simulink library "DCL"  (R2018b)
settings: Solver=VariableStepAuto  StartTime=0.0  StopTime=10.0  RelTol=1e-3
undefined symbols (not defined in the file or in its folder): Uc_max, Uc_min
libraries: simulink x11
settings Model: Creator=a0741273  LastModifiedBy=a0741273
settings SFSimCC: SimUseLocalCustomCode=off
settings RTWCC: RTWUseLocalCustomCode=off

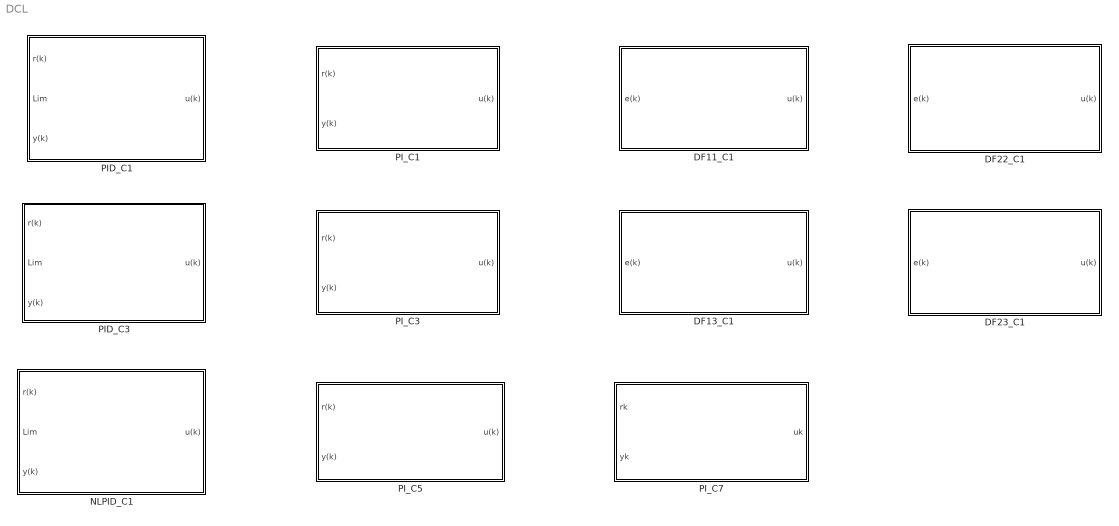
== system DCL ==
  DF11_C1 : Subsystem  TreatAsAtomicUnit=on  SystemSampleTime=T  mask{b0=1, b1=0, a1=0, T=0.001}
      mask prompts: b0 "Coefficient b0"; b1 "Coefficient b1"; a1 "Coefficient a1"; T "Sample period in seconds"
      mask Help:
      | The DF11_C1 block provides a functional model of a first order discrete "direct form 1" compensator in the C2000 Digital Control Library (DCL).
      | 
      | The control law is:
      | u(k) = b0*e(k) + b1*e(k-1) - a1*u(k-1)
      | 
      | T = The sample period (controller update rate) in seconds.
      | 
      | Refer to the DCL User's Guide for further information about this controller.  The model is not configured to support code generation.
      mask DialogControl DescTextVar Prompt: DF11_C1 Controller Parameters
      mask Display: disp('DF11_C1')
  DF13_C1 : Subsystem  TreatAsAtomicUnit=on  mask{b0=1, b1=0, b2=0, b3=0, a1=0, a2=0, a3=0, T=0.001}
      mask prompts: b0 "Coefficient b0"; b1 "Coefficient b1"; b2 "Coefficient b2"; b3 "Coefficient b3"; a1 "Coefficient a1"; a2 "Coefficient a2"; a3 "Coefficient a3"; T "Sample period in seconds"
      mask Help:
      | The DF13_C1 block provides a functional model of a third order discrete "direct form 1" compensator in the C2000 Digital Control Library (DCL).
      | 
      | The control law is:
      | u(k) = b0*e(k) + b1*e(k-1) + b2*e(k-2) + b3*e(k-3) - a1*u(k-1) - a2*u(k-2) - a3*u(k-3)
      | 
      | T = The sample period (controller update rate) in seconds.
      | 
      | Refer to the DCL User's Guide for further information about this controller.  The model is not configured to support code generation.
      mask DialogControl DescTextVar Prompt: DF13_C1 Controller Parameters
      mask DialogControl T Tooltip: Enter sample period in seconds
      mask Display: disp('DF13_C1')
  DF22_C1 : Subsystem  TreatAsAtomicUnit=on  SystemSampleTime=T  mask{b0=1, b1=0, b2=0, a1=0, a2=0, T=0.001}
      mask prompts: b0 "Coefficient b0"; b1 "Coefficient b1"; b2 "Coefficient b2"; a1 "Coefficient a1"; a2 "Coefficient a2"; T "Sample period in seconds"
      mask Help:
      | The DF22_C1 block provides a functional model of a second order discrete "direct form 2" compensator in the C2000 Digital Control Library (DCL).
      | 
      | The control law is:
      | u(k) = b0*e(k) + b1*e(k-1) + b2*e(k-2) - a1*u(k-1) - a2*u(k-2)
      | 
      | T = The sample period (controller update rate) in seconds.
      | 
      | Refer to the DCL User's Guide for further information about this controller.  The model is not configured to support code generation.
      mask DialogControl DescTextVar Prompt: CF22_C1 Controller Parameters
      mask Display: disp('DF22_C1')
  DF23_C1 : Subsystem  TreatAsAtomicUnit=on  mask{b0=1, b1=0, b2=0, b3=0, a1=0, a2=0, a3=0, T=0.001}
      mask prompts: b0 "Coefficient b0"; b1 "Coefficient b1"; b2 "Coefficient b2"; b3 "Coefficient b3"; a1 "Coefficient a1"; a2 "Coefficient a2"; a3 "Coefficient a3"; T "Sample period in seconds"
      mask Help:
      | he DF23_C1 block provides a functional model of a third order discrete "direct form 2" compensator in the C2000 Digital Control Library (DCL).
      | 
      | The control law is:
      | u(k) = b0*e(k) + b1*e(k-1) + b2*e(k-2) + b3*e(k-3) - a1*u(k-1) - a2*u(k-2) - a3*u(k-3)
      | 
      | T = The sample period (controller update rate) in seconds.
      | 
      | Refer to the DCL User's Guide for further information about this controller.  The model is not configured to support code generation.
      mask DialogControl DescTextVar Prompt: DF23_C1 Controller Parameters
      mask Display: disp('DF23_C1')
  NLPID_C1 : Subsystem  TreatAsAtomicUnit=on  SystemSampleTime=T  mask{Kp=1, Ki=0, Kd=0, alpha_p=1, alpha_i=1, alpha_d=1, delta_p=0.1, delta_i=0.1, delta_d=0.1, fc=100, Umax=1, Umin=-1, T=0.001}
      mask prompts: Kp "Linear Proportional Gain (Kp)"; Ki "Linear Integral Gain (Ki)"; Kd "Linear Derivative Gain (Kd)"; alpha_p "P-path Non-linear Coefficient (alpha_p)"; alpha_i "I-path Non-linear Coefficient (alpha_i)"; alpha_d "D-path Non-linear Coefficient (alpha_d)"; delta_p "P-path Linear Semi-width (delta_p)"; delta_i "I-path Linear Semi-width (delta_i)"; delta_d "D-path Linear Semi-width (delta_d)"; fc "Derivative Filter Bandwidth in Hz"; Umax "Output Clamp Upper Limit (Umax)"; Umin "Output Clamp Lower Limit (Umin)"; T "Sample Period in seconds"
      mask help: C2000 Digital Control Library blocks
      mask init:
      | tau = 1 / (2*pi*fc);
      | c1 = 2 / (T + 2*tau);
      | c2 = (T - 2*tau) / (T + 2*tau);
      | 
      | gamma_p = 1 / (delta_p^(1 - alpha_p));
      | gamma_i = 1 / (delta_i^(1 - alpha_i));
      | gamma_d = 1 / (delta_d^(1 - alpha_d));
      mask Help:
      | The NLPID_C1 block provides a functional model of the non-linear PID controller in the C2000 Digital Control Library (DCL).
      | 
      | Kp = Linear proportional gain
      | Ki = Linear integral gain
      | Kd = Linear derivative gain
      | alpha_p = P-path non-linear exponent
      | alpha_i = I-path non-linear exponent
      | alpha_d = D-path non-linear exponent
      | delta_p = P-path linearized semi-width
      | delta_i = I-path linearized semi-width
      | delta_d = D-path linearized semi-width
      | Umax = Output clamp upper limit
      | Umin = Output clamp lower limit
      | 
      | Refer to the DCL User's Guide for further information on this controller.  The model is not configured to support code generation.
      mask DialogControl DescTextVar Prompt: NLPID_C1 Controller Parameters
      mask Display:
      | disp('NLPID_C1')
      | % image('C:\Aa07\projects\DCL\models\SLOGO.jpg')
  PID_C1 : Subsystem  TreatAsAtomicUnit=on  SystemSampleTime=T  mask{Kp=1, Ki=0, Kd=0, Kr=1, fc=100, Umax=1, Umin=-1, T=0.001}
      mask prompts: Kp "Proportional Gain (Kp)"; Ki "Integral Gain (Ki)"; Kd "Derivative Gain (Kd)"; Kr "Set-point Gain (Kr)"; fc "Derivative Filter Bandwidth in Hz (fc)"; Umax "Output Clamp Upper Limit (Umax)"; Umin "Output Clamp Lower Limit (Umin)"; T "Sample Period in seconds (T)"
      mask init:
      | tau = 1 / (2*pi*fc);
      | c1 = 2 / (T + 2*tau);
      | c2 = (T - 2*tau) / (T + 2*tau);
      mask Help:
      | The PID_C1 block provides a functional model of the series form linear PID controller in the C2000 Digital Control Library (DCL).
      | 
      | Kp = The proportional path gain.
      | 
      | Ki = The integral path gain scaled by the sample period (T).
      | 
      | Kd = The derivative path gain.  Sample period enters the control law through the derivative filter coefficients, so is not accounted for in Kd.
      | 
      | Kr = The set-point weighting factor.
      | 
      | fc = The -3dB bandwidth of the derivative filter in Hz.  This is used to compute the derivative filter coefficients c1 & c2.
      | 
      | Umax = The upper limit of the output clamp.
      | 
      | Umin = The lower limit of the output clamp.
      | 
      | T = The sample period (controller update rate) in seconds.
      | 
      | Refer to the DCL User's Guide for further information about this controller.  The model is not configured to support code generation.
      mask DialogControl DescTextVar Prompt: PID_C1 Controller Parameters
      mask Display: disp('PID_C1')
  PID_C3 : Subsystem  TreatAsAtomicUnit=on  SystemSampleTime=T  mask{Kp=1, Ki=0, Kd=0, fc=100, Umax=1, Umin=-1, T=0.001}
      mask prompts: Kp "Proportional Gain (Kp)"; Ki "Integral Gain (Ki)"; Kd "Derivative Gain (Kd)"; fc "Derivative Filter Bandwidth in Hz (fc)"; Umax "Output Clamp Upper Limit (Umax)"; Umin "Output Clamp Lower Limit (Umin)"; T "Sample Period in seconds (T)"
      mask init:
      | tau = 1 / (2*pi*fc);
      | c1 = 2 / (T + 2*tau);
      | c2 = (T - 2*tau) / (T + 2*tau);
      mask Help:
      | The PID_C3 block provides a functional model of the parallel form linear PID controller in the C2000 Digital Control Library (DCL).
      | 
      | Kp = The proportional path gain.
      | 
      | Ki = The integral path gain scaled by the sample period (T).
      | 
      | Kd = The derivative path gain.  Sample period enters the control law through the derivative filter coefficients, so is not accounted for in Kd.
      | 
      | fc = The -3dB bandwidth of the derivative filter in Hz.  This is used to compute the derivative filter coefficients c1 & c2.
      | 
      | Umax = The upper limit of the output clamp.
      | 
      | Umin = The lower limit of the output clamp.
      | 
      | T = The sample period (controller update rate) in seconds.
      | 
      | Refer to the DCL User's Guide for further information about this controller.  The model is not configured to support code generation.
      mask DialogControl DescTextVar Prompt: PID_C3 Controller Parameters
      mask Display: disp('PID_C3')
  PI_C1 : Subsystem  TreatAsAtomicUnit=on  SystemSampleTime=T  mask{Kp=1, Ki=0, Umax=1, Umin=-1, T=0.001}
      mask prompts: Kp "Proportional Gain (Kp)"; Ki "Integral Gain (Ki)"; Umax "Output Clamp Upper Limit (Umax)"; Umin "Output Clamp Upper Limit (Umin)"; T "Sample period in seconds"
      mask Help:
      | The PI_C1 block provides a functional model of the series form linear PI controller in the C2000 Digital Control Library (DCL).
      | 
      | Kp = The proportional path gain.
      | 
      | Ki = The integral path gain scaled by the sample period (T).
      | 
      | Umax = The upper limit of the output clamp.
      | 
      | Umin = The lower limit of the output clamp.
      | 
      | T = The sample period (controller update rate) in seconds.
      | 
      | Refer to the DCL User's Guide for further information about this controller.  The model is not configured to support code generation.
      mask DialogControl DescTextVar Prompt: PI_C3 Controller Parameters
      mask Display: disp('PI_C1')
  PI_C3 : Subsystem  TreatAsAtomicUnit=on  SystemSampleTime=T  mask{Kp=1, Ki=0, Umax=1, Umin=-1, T=0.001}
      mask prompts: Kp "Proportional Gain (Kp)"; Ki "Integral Gain (Ki)"; Umax "Output Clamp Upper Limit (Umax)"; Umin "Output Clamp Lower Limit (Umin)"; T "Sample period in seconds"
      mask Help:
      | The PI_C3 block provides a functional model of the parallel form linear PI controller in the C2000 Digital Control Library (DCL).
      | 
      | Kp = The proportional path gain.
      | 
      | Ki = The integral path gain scaled by the sample period (T).
      | 
      | Umax = The upper limit of the output clamp.
      | 
      | Umin = The lower limit of the output clamp.
      | 
      | T = The sample period (controller update rate) in seconds.
      | 
      | Refer to the DCL User's Guide for further information about this controller.  The model is not configured to support code generation.
      mask DialogControl DescTextVar Prompt: PI_C3 Controller Parameters
      mask Display: disp('PI_C3')
  PI_C5 : Subsystem  TreatAsAtomicUnit=on  SystemSampleTime=T  mask{Kp=1, Ki=0, Umax=1, Umin=-1, Imax=1, Imin=-1, T=0.001}
      mask prompts: Kp "Proportional Gain (Kp)"; Ki "Integral Gain (Ki)"; Umax "Output Clamp Upper Limit (Umax)"; Umin "Output Clamp Lower Limit (Umin)"; Imax "Integrator Clamp Upper Limit (Imax)"; Imin "Integrator Clamp Lower Limit (Imin)"; T "Sample period in seconds"
      mask Help:
      | The PI_C5 block provides a functional model of the parallel form linear PI controller in the C2000 Digital Control Library (DCL).  This controller comprises separate integral path and output clamp limits and employs improved, though less cycle efficient, anti-windup reset logic.
      | 
      | Kp = The proportional path gain.
      | 
      | Ki = The integral path gain scaled by the sample period (T).
      | 
      | Umax = The upper limit of the output clamp.
      | 
      | Umin = The lower limit of the output clamp.
      | 
      | Imax = The upper limit of the integrator clamp.
      | 
      | Imin = The lower limit of the integrator clamp.
      | 
      | T = The sample period (controller update rate) in seconds.
      | 
      | Refer to the DCL User's Guide for further information about this controller.  The model is not configured to support code generation.
      mask DialogControl DescTextVar Prompt: PI_C5 Controller Parameters
      mask Display: disp('PI_C5')
  PI_C7 : Subsystem  mask{Kp=1, Ki=0, Umax=1, Umin=-1, T=0.001}
      mask prompts: Kp "Proportional Gain (Kp)"; Ki "Integral Gain (Ki)"; Umax "Output clamp Upper Limit (Umax)"; Umin "Output Clamp Lower Limit (Umin)"; T "Sample Rate in Seconds"
      mask Help:
      | The PI_C7 block provides a functional model of the series form linear PI controller with Tustin integrator in the C2000 Digital Control Library (DCL).  The model is functionally similar to the PI_C6 and PI_C7 controllers.
      | 
      | Kp = The proportional path gain.
      | 
      | Ki = The integral path gain scaled by the sample period (T).
      | 
      | Umax = The upper limit of the output clamp.
      | 
      | Umin = The lower limit of the output clamp.
      | 
      | T = The sample period (controller update rate) in seconds.
      | 
      | Refer to the DCL User's Guide for further information about this controller.  The model is not configured to support code generation.
      mask DialogControl DescTextVar Prompt: PI_C7 Controller Parameters
      mask Display: disp('PI_C7')

== system DCL/DF11_C1 ==
  e(k) : Inport
  Gain : Gain  Gain=b0
  Gain1 : Gain  Gain=b1
  Gain2 : Gain  Gain=a1
  Sum : Sum  Inputs=+|-
  Sum1 : Sum  Inputs=++|
  Unit Delay : UnitDelay  SampleTime=-1
  Unit Delay5 : UnitDelay  SampleTime=-1
  u(k) : Outport
  wires:
  Gain/1 -> Sum/1
  Unit Delay/1 -> Gain1/1
  e(k)/1 -> Gain/1, Unit Delay/1
  Unit Delay5/1 -> Gain2/1
  Gain1/1 -> Sum1/1
  Sum/1 -> Sum1/2
  Sum1/1 -> Unit Delay5/1, u(k)/1
  Gain2/1 -> Sum/2

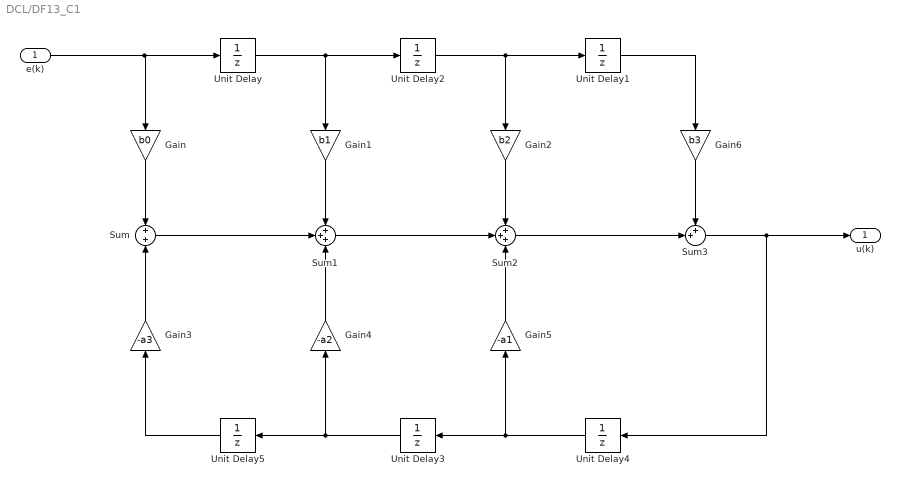
== system DCL/DF13_C1 ==
  e(k) : Inport
  Gain : Gain  Gain=b0
  Gain1 : Gain  Gain=b1
  Gain2 : Gain  Gain=b2
  Gain3 : Gain  Gain=-a3
  Gain4 : Gain  Gain=-a2
  Gain5 : Gain  Gain=-a1
  Gain6 : Gain  Gain=b3
  Sum : Sum  Inputs=+|+
  Sum1 : Sum  Inputs=+++
  Sum2 : Sum  Inputs=+++
  Sum3 : Sum  Inputs=++|
  Unit Delay{,1..5} (6 alike) : UnitDelay  SampleTime=-1
  "u(k) " : Outport
  wires:
  e(k)/1 -> Gain/1, Unit Delay/1
  Unit Delay/1 -> Gain1/1, Unit Delay2/1
  Unit Delay2/1 -> Gain2/1, Unit Delay1/1
  Unit Delay4/1 -> Gain5/1, Unit Delay3/1
  Unit Delay3/1 -> Gain4/1, Unit Delay5/1
  Gain/1 -> Sum/1
  Gain1/1 -> Sum1/1
  Gain2/1 -> Sum2/1
  Sum/1 -> Sum1/2
  Sum1/1 -> Sum2/2
  Gain3/1 -> Sum/2
  Gain4/1 -> Sum1/3
  Gain5/1 -> Sum2/3
  Unit Delay1/1 -> Gain6/1
  Gain6/1 -> Sum3/1
  Sum2/1 -> Sum3/2
  Unit Delay5/1 -> Gain3/1
  Sum3/1 -> "u(k) "/1, Unit Delay4/1

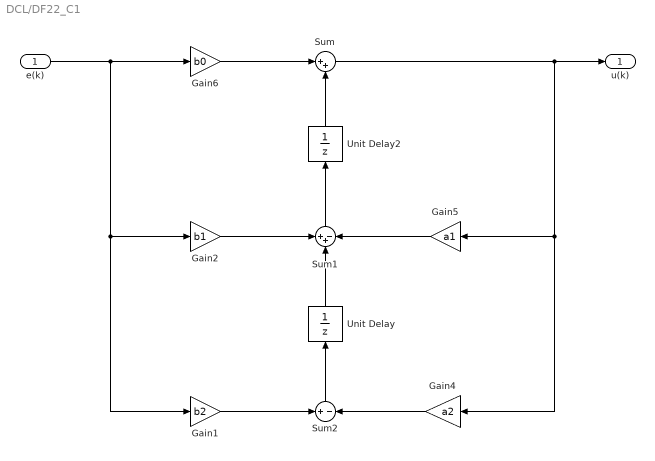
== system DCL/DF22_C1 ==
  e(k) : Inport
  Gain1 : Gain  Gain=b2
  Gain2 : Gain  Gain=b1
  Gain4 : Gain  Gain=a2
  Gain5 : Gain  Gain=a1
  Gain6 : Gain  Gain=b0
  Sum : Sum  Inputs=|++
  Sum1 : Sum  Inputs=++-
  Sum2 : Sum  Inputs=+|-
  Unit Delay : UnitDelay  SampleTime=-1
  Unit Delay2 : UnitDelay  SampleTime=-1
  "u(k) " : Outport
  wires:
  Gain2/1 -> Sum1/1
  Unit Delay/1 -> Sum1/2
  Sum1/1 -> Unit Delay2/1
  Unit Delay2/1 -> Sum/2
  Gain5/1 -> Sum1/3
  Gain4/1 -> Sum2/2
  Sum2/1 -> Unit Delay/1
  Gain1/1 -> Sum2/1
  e(k)/1 -> Gain2/1, Gain1/1, Gain6/1
  Gain6/1 -> Sum/1
  Sum/1 -> Gain4/1, Gain5/1, "u(k) "/1

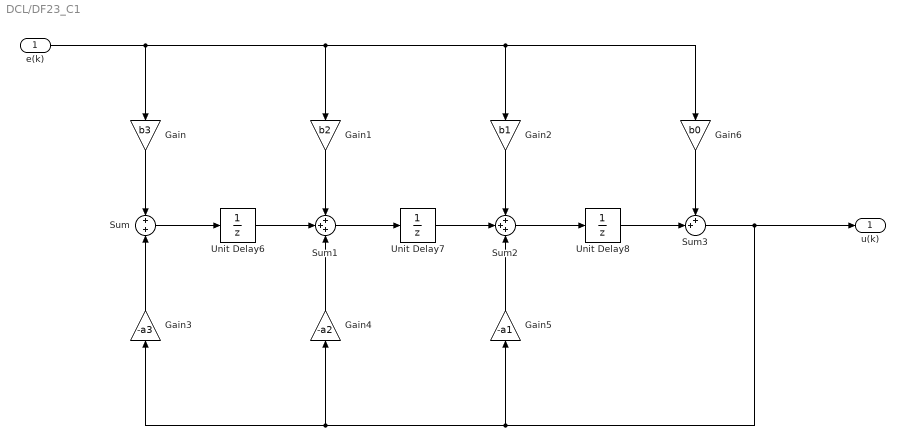
== system DCL/DF23_C1 ==
  e(k) : Inport
  Gain : Gain  Gain=b3
  Gain1 : Gain  Gain=b2
  Gain2 : Gain  Gain=b1
  Gain3 : Gain  Gain=-a3
  Gain4 : Gain  Gain=-a2
  Gain5 : Gain  Gain=-a1
  Gain6 : Gain  Gain=b0
  Sum : Sum  Inputs=+|+
  Sum1 : Sum  Inputs=+++
  Sum2 : Sum  Inputs=+++
  Sum3 : Sum  Inputs=++|
  Unit Delay6 : UnitDelay  SampleTime=-1
  Unit Delay7 : UnitDelay  SampleTime=-1
  Unit Delay8 : UnitDelay  SampleTime=-1
  "u(k) " : Outport
  wires:
  Gain/1 -> Sum/1
  Gain1/1 -> Sum1/1
  Gain2/1 -> Sum2/1
  Gain3/1 -> Sum/2
  Gain4/1 -> Sum1/3
  Gain5/1 -> Sum2/3
  e(k)/1 -> Gain/1, Gain6/1, Gain2/1, Gain1/1
  Gain6/1 -> Sum3/1
  Sum3/1 -> Gain3/1, Gain4/1, Gain5/1, "u(k) "/1
  Unit Delay8/1 -> Sum3/2
  Sum2/1 -> Unit Delay8/1
  Unit Delay7/1 -> Sum2/2
  Sum1/1 -> Unit Delay7/1
  Unit Delay6/1 -> Sum1/2
  Sum/1 -> Unit Delay6/1

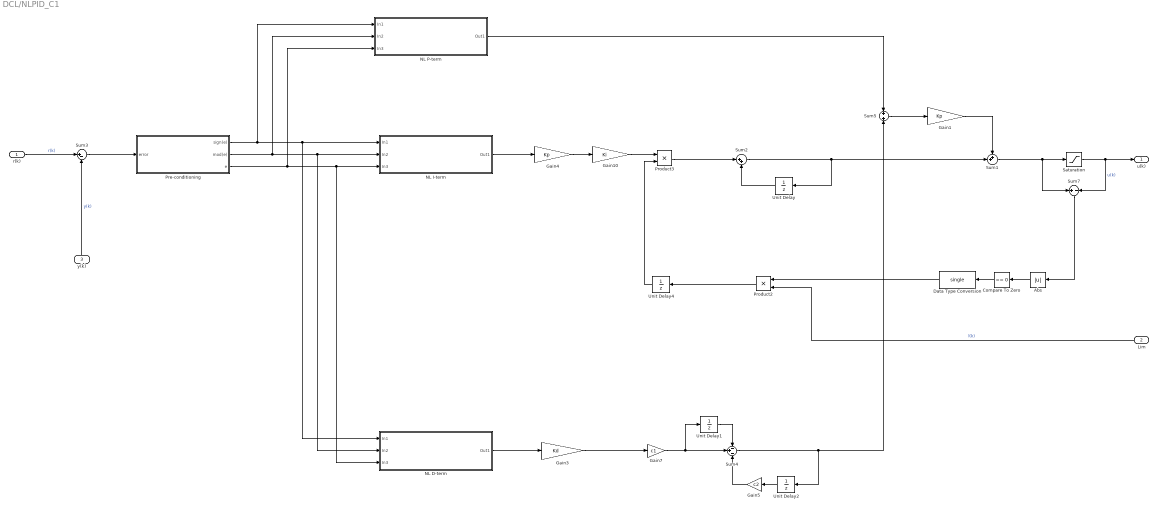
== system DCL/NLPID_C1 ==
  r(k) : Inport  OutDataTypeStr=single  SampleTime=T
  Lim : Inport  Port=2  OutDataTypeStr=single  SampleTime=T  LockScale=on
  y(k) : Inport  Port=3  OutDataTypeStr=single  SampleTime=T  LockScale=on
  Abs : Abs
  Compare To Zero : simulink/Logic and Bit Operations/Compare To Zero  relop===  OutDataTypeStr=boolean
  Data Type Conversion : DataTypeConversion  OutDataTypeStr=single
  Gain1 : Gain  Gain=Kp
  Gain10 : Gain  Gain=Ki
  Gain3 : Gain  Gain=Kd
  Gain4 : Gain  Gain=Kp
  Gain5 : Gain  Gain=c2  ParamDataTypeStr=single  OutDataTypeStr=single  LockScale=on
  Gain7 : Gain  Gain=c1
  NL D-term : Subsystem
  NL I-term : Subsystem
  NL P-term : Subsystem
  Pre-conditioning : Subsystem
  Product2 : Product  RndMeth=Zero
  Product3 : Product  RndMeth=Zero
  Saturation : Saturate  UpperLimit=Umax  LowerLimit=Umin
  Sum1 : Sum  Inputs=++|
  Sum2 : Sum  Inputs=|++
  Sum3 : Sum  Inputs=|+-  AccumDataTypeStr=single  OutDataTypeStr=single  InputSameDT=on  LockScale=on
  Sum4 : Sum  Inputs=-+-
  Sum5 : Sum  Inputs=+|+
  Sum7 : Sum  Inputs=+|-
  Unit Delay{,1..2,4} (4 alike) : UnitDelay  SampleTime=-1
  u(k) : Outport
  wires:
  Sum5/1 -> Gain1/1
  Gain1/1 -> Sum1/1
  Gain4/1 -> Gain10/1
  Gain10/1 -> Product3/1
  Gain3/1 -> Gain7/1
  Sum4/1 -> Unit Delay2/1, Sum5/2
  NL P-term/1(Out1) -> Sum5/1
  Sum1/1 -> Saturation/1, Sum7/1
  Sum7/1 -> Abs/1
  NL D-term/1(Out1) -> Gain3/1
  NL I-term/1(Out1) -> Gain4/1
  Pre-conditioning/3(e) -> NL I-term/3(In3), NL D-term/3(In3), NL P-term/3(In3)
  Pre-conditioning/2(mod(e)) -> NL I-term/2(In2), NL D-term/2(In2), NL P-term/2(In2)
  Pre-conditioning/1(sign(e)) -> NL I-term/1(In1), NL D-term/1(In1), NL P-term/1(In1)
  Sum3/1 -> Pre-conditioning/1(error)
  Unit Delay4/1 -> Product3/2
  Lim/1 -> Product2/2  "l(k)"
  Product3/1 -> Sum2/1
  Compare To Zero/1 -> Data Type Conversion/1
  Product2/1 -> Unit Delay4/1
  Data Type Conversion/1 -> Product2/1
  Saturation/1 -> u(k)/1, Sum7/2  "u(k)"
  Abs/1 -> Compare To Zero/1
  Sum2/1 -> Sum1/2, Unit Delay/1
  Unit Delay/1 -> Sum2/2
  Gain5/1 -> Sum4/3
  Unit Delay2/1 -> Gain5/1
  Unit Delay1/1 -> Sum4/1
  Gain7/1 -> Sum4/2, Unit Delay1/1
  y(k)/1 -> Sum3/2  "y(k)"
  r(k)/1 -> Sum3/1  "r(k)"

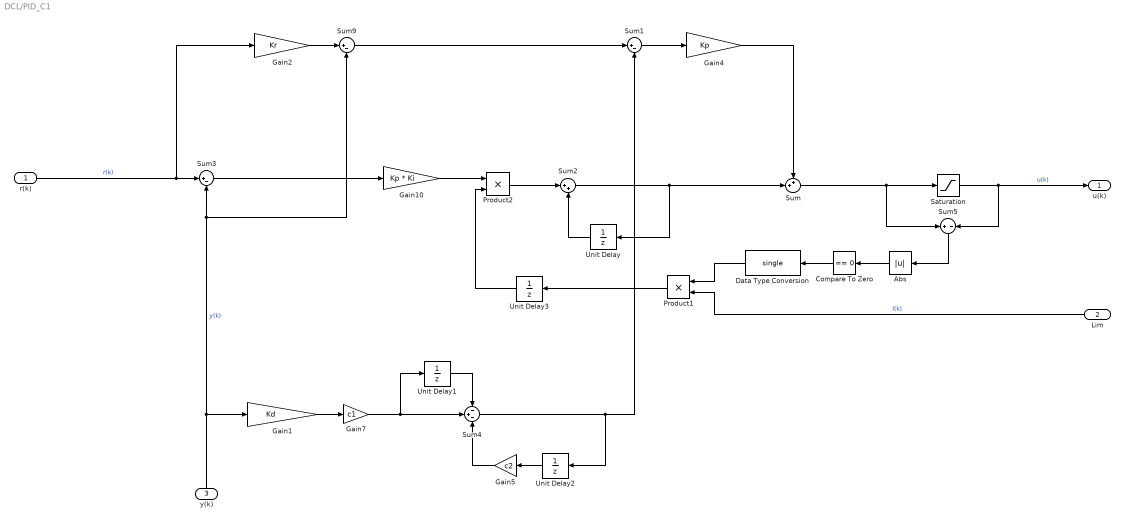
== system DCL/PID_C1 ==
  r(k) : Inport  OutDataTypeStr=single  SampleTime=T  LockScale=on
  Lim : Inport  Port=2  OutDataTypeStr=single  SampleTime=T  LockScale=on
  y(k) : Inport  Port=3  OutDataTypeStr=single  SampleTime=T
  Abs : Abs
  Compare To Zero : simulink/Logic and Bit Operations/Compare To Zero  relop===  OutDataTypeStr=boolean
  Data Type Conversion : DataTypeConversion  OutDataTypeStr=single
  Gain1 : Gain  Gain=Kd
  Gain10 : Gain  Gain=Kp * Ki
  Gain2 : Gain  Gain=Kr
  Gain4 : Gain  Gain=Kp
  Gain5 : Gain  Gain=c2
  Gain7 : Gain  Gain=c1
  Product1 : Product  RndMeth=Zero
  Product2 : Product  RndMeth=Zero
  Saturation : Saturate  UpperLimit=Umax  LowerLimit=Umin
  Sum : Sum  Inputs=++|
  Sum1 : Sum  Inputs=|+-
  Sum2 : Sum  Inputs=|++
  Sum3 : Sum  Inputs=|+-
  Sum4 : Sum  Inputs=-+-
  Sum5 : Sum  Inputs=+|-
  Sum9 : Sum  Inputs=|+-
  Unit Delay{,1..3} (4 alike) : UnitDelay  SampleTime=-1
  u(k) : Outport
  wires:
  Unit Delay/1 -> Sum2/2
  Sum/1 -> Sum5/1, Saturation/1
  Gain5/1 -> Sum4/3
  Unit Delay2/1 -> Gain5/1
  Unit Delay1/1 -> Sum4/1
  Gain1/1 -> Gain7/1
  Gain7/1 -> Sum4/2, Unit Delay1/1
  Gain10/1 -> Product2/1
  Sum3/1 -> Gain10/1
  Sum1/1 -> Gain4/1
  Gain4/1 -> Sum/1
  Sum2/1 -> Unit Delay/1, Sum/2
  Gain2/1 -> Sum9/1
  Sum9/1 -> Sum1/1
  Sum4/1 -> Unit Delay2/1, Sum1/2
  r(k)/1 -> Gain2/1, Sum3/1  "r(k)"
  y(k)/1 -> Sum9/2, Sum3/2, Gain1/1  "y(k)"
  Lim/1 -> Product1/2  "l(k)"
  Product2/1 -> Sum2/1
  Saturation/1 -> Sum5/2, u(k)/1  "u(k)"
  Sum5/1 -> Abs/1
  Abs/1 -> Compare To Zero/1
  Compare To Zero/1 -> Data Type Conversion/1
  Data Type Conversion/1 -> Product1/1
  Product1/1 -> Unit Delay3/1
  Unit Delay3/1 -> Product2/2

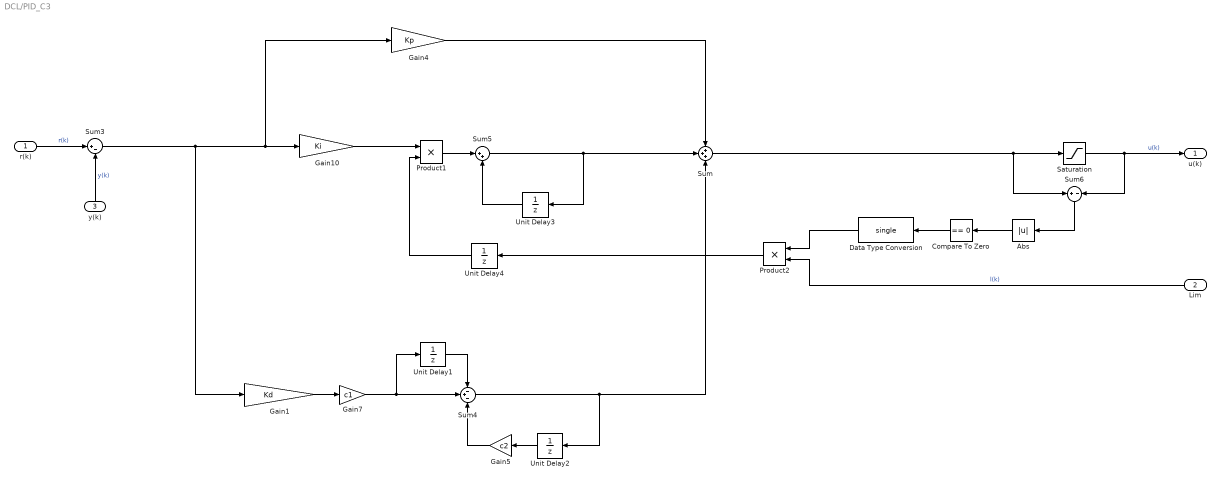
== system DCL/PID_C3 ==
  r(k) : Inport  OutDataTypeStr=single  SampleTime=T  LockScale=on
  Lim : Inport  Port=2  SampleTime=T  LockScale=on
  y(k) : Inport  Port=3  OutDataTypeStr=single  SampleTime=T  LockScale=on
  Abs : Abs
  Compare To Zero : simulink/Logic and Bit Operations/Compare To Zero  relop===  OutDataTypeStr=boolean
  Data Type Conversion : DataTypeConversion  OutDataTypeStr=single
  Gain1 : Gain  Gain=Kd
  Gain10 : Gain  Gain=Ki
  Gain4 : Gain  Gain=Kp
  Gain5 : Gain  Gain=c2
  Gain7 : Gain  Gain=c1
  Product1 : Product  RndMeth=Zero
  Product2 : Product  RndMeth=Zero
  Saturation : Saturate  UpperLimit=Umax  LowerLimit=Umin
  Sum : Sum  Inputs=+++
  Sum3 : Sum  Inputs=|+-
  Sum4 : Sum  Inputs=-+-
  Sum5 : Sum  Inputs=|++
  Sum6 : Sum  Inputs=+|-
  Unit Delay{1..4} (4 alike) : UnitDelay  SampleTime=-1
  u(k) : Outport
  wires:
  r(k)/1 -> Sum3/1  "r(k)"
  Sum4/1 -> Sum/3, Unit Delay2/1
  Gain4/1 -> Sum/1
  Sum3/1 -> Gain1/1, Gain4/1, Gain10/1
  Gain7/1 -> Unit Delay1/1, Sum4/2
  Gain1/1 -> Gain7/1
  Unit Delay1/1 -> Sum4/1
  Unit Delay2/1 -> Gain5/1
  Gain5/1 -> Sum4/3
  y(k)/1 -> Sum3/2  "y(k)"
  Unit Delay3/1 -> Sum5/2
  Sum/1 -> Sum6/1, Saturation/1
  Sum5/1 -> Sum/2, Unit Delay3/1
  Saturation/1 -> u(k)/1, Sum6/2  "u(k)"
  Sum6/1 -> Abs/1
  Abs/1 -> Compare To Zero/1
  Compare To Zero/1 -> Data Type Conversion/1
  Data Type Conversion/1 -> Product2/1
  Product2/1 -> Unit Delay4/1
  Lim/1 -> Product2/2  "l(k)"
  Product1/1 -> Sum5/1
  Unit Delay4/1 -> Product1/2
  Gain10/1 -> Product1/1

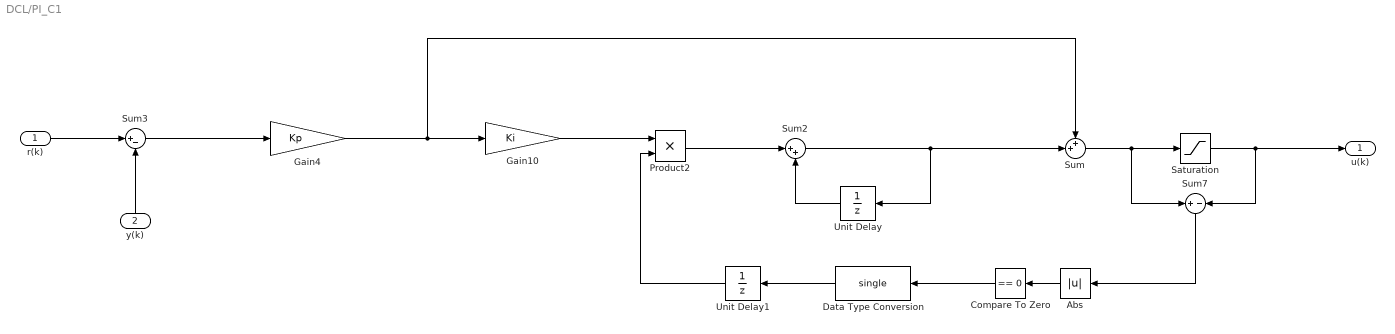
== system DCL/PI_C1 ==
  r(k) : Inport
  y(k) : Inport  Port=2
  Abs : Abs
  Compare To Zero : simulink/Logic and Bit Operations/Compare To Zero  relop===  OutDataTypeStr=uint8  ZeroCross=off
  Data Type Conversion : DataTypeConversion  OutDataTypeStr=single
  Gain10 : Gain  Gain=Ki
  Gain4 : Gain  Gain=Kp
  Product2 : Product  RndMeth=Zero
  Saturation : Saturate  UpperLimit=Umax  LowerLimit=Umin
  Sum : Sum  Inputs=++|
  Sum2 : Sum  Inputs=|++
  Sum3 : Sum  Inputs=|+-
  Sum7 : Sum  Inputs=+|-
  Unit Delay : UnitDelay  SampleTime=-1
  Unit Delay1 : UnitDelay  SampleTime=-1
  u(k) : Outport
  wires:
  Unit Delay/1 -> Sum2/2
  Gain10/1 -> Product2/1
  Sum3/1 -> Gain4/1
  Sum2/1 -> Unit Delay/1, Sum/2
  r(k)/1 -> Sum3/1
  y(k)/1 -> Sum3/2
  Gain4/1 -> Sum/1, Gain10/1
  Sum7/1 -> Abs/1
  Saturation/1 -> u(k)/1, Sum7/2
  Sum/1 -> Sum7/1, Saturation/1
  Abs/1 -> Compare To Zero/1
  Compare To Zero/1 -> Data Type Conversion/1
  Product2/1 -> Sum2/1
  Data Type Conversion/1 -> Unit Delay1/1
  Unit Delay1/1 -> Product2/2

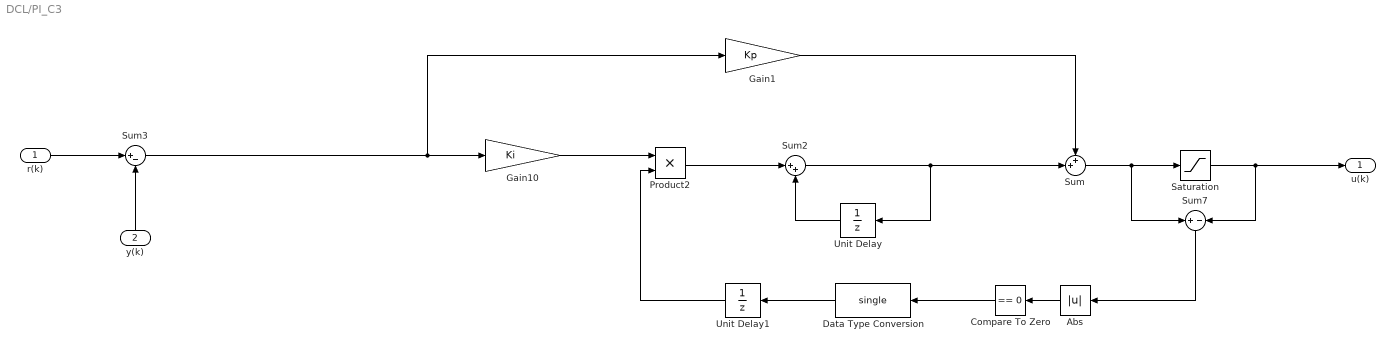
== system DCL/PI_C3 ==
  r(k) : Inport
  y(k) : Inport  Port=2
  Abs : Abs
  Compare To Zero : simulink/Logic and Bit Operations/Compare To Zero  relop===  OutDataTypeStr=uint8  ZeroCross=off
  Data Type Conversion : DataTypeConversion  OutDataTypeStr=single
  Gain1 : Gain  Gain=Kp
  Gain10 : Gain  Gain=Ki
  Product2 : Product  RndMeth=Zero
  Saturation : Saturate  UpperLimit=Umax  LowerLimit=Umin
  Sum : Sum  Inputs=++|
  Sum2 : Sum  Inputs=|++
  Sum3 : Sum  Inputs=|+-
  Sum7 : Sum  Inputs=+|-
  Unit Delay : UnitDelay  SampleTime=-1
  Unit Delay1 : UnitDelay  SampleTime=-1
  u(k) : Outport
  wires:
  Unit Delay/1 -> Sum2/2
  Gain10/1 -> Product2/1
  Sum2/1 -> Unit Delay/1, Sum/2
  r(k)/1 -> Sum3/1
  y(k)/1 -> Sum3/2
  Sum3/1 -> Gain1/1, Gain10/1
  Sum7/1 -> Abs/1
  Saturation/1 -> u(k)/1, Sum7/2
  Sum/1 -> Sum7/1, Saturation/1
  Abs/1 -> Compare To Zero/1
  Compare To Zero/1 -> Data Type Conversion/1
  Product2/1 -> Sum2/1
  Data Type Conversion/1 -> Unit Delay1/1
  Unit Delay1/1 -> Product2/2
  Gain1/1 -> Sum/1

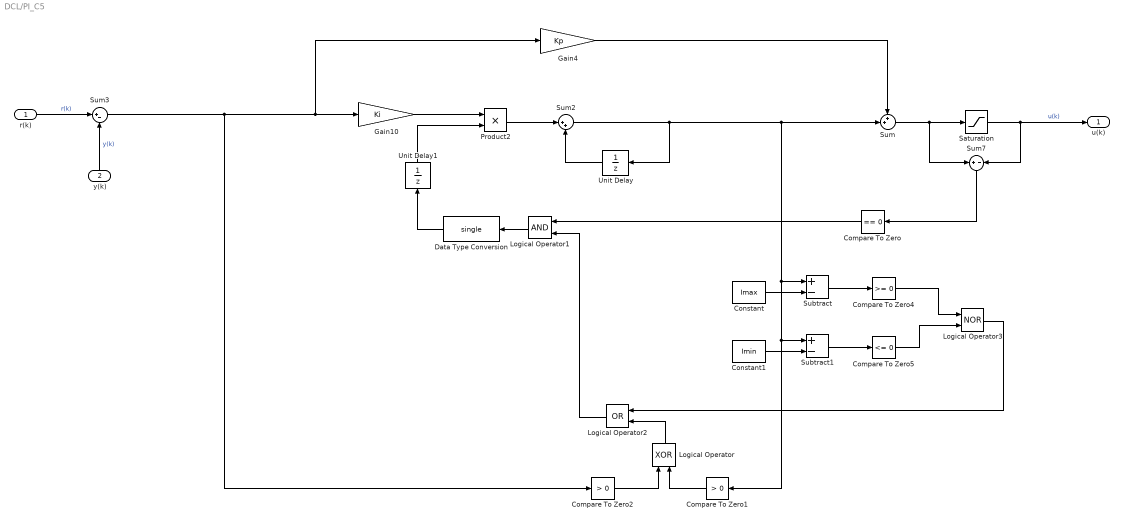
== system DCL/PI_C5 ==
  r(k) : Inport
  y(k) : Inport  Port=2
  Compare To Zero : simulink/Logic and Bit Operations/Compare To Zero  relop===  OutDataTypeStr=boolean  ZeroCross=off
  Compare To Zero1 : simulink/Logic and Bit Operations/Compare To Zero  relop=>  OutDataTypeStr=boolean  ZeroCross=off
  Compare To Zero2 : simulink/Logic and Bit Operations/Compare To Zero  relop=>  OutDataTypeStr=boolean  ZeroCross=off
  Compare To Zero4 : simulink/Logic and Bit Operations/Compare To Zero  relop=>=  OutDataTypeStr=boolean  ZeroCross=off
  Compare To Zero5 : simulink/Logic and Bit Operations/Compare To Zero  relop=<=  OutDataTypeStr=boolean  ZeroCross=off
  Constant : Constant  Value=Imax  SampleTime=T
  Constant1 : Constant  Value=Imin  SampleTime=T
  Data Type Conversion : DataTypeConversion  OutDataTypeStr=single
  Gain10 : Gain  Gain=Ki
  Gain4 : Gain  Gain=Kp
  Logical Operator : Logic  Operator=XOR  AllPortsSameDT=off  OutDataTypeStr=boolean
  Logical Operator1 : Logic  AllPortsSameDT=off  OutDataTypeStr=boolean
  Logical Operator2 : Logic  Operator=OR  AllPortsSameDT=off  OutDataTypeStr=boolean
  Logical Operator3 : Logic  Operator=NOR  AllPortsSameDT=off  OutDataTypeStr=boolean
  Product2 : Product  RndMeth=Zero
  Saturation : Saturate  UpperLimit=Umax  LowerLimit=Umin
  Subtract : Sum  Inputs=+-
  Subtract1 : Sum  Inputs=+-
  Sum : Sum  Inputs=++|
  Sum2 : Sum  Inputs=|++
  Sum3 : Sum  Inputs=|+-
  Sum7 : Sum  Inputs=+|-
  Unit Delay : UnitDelay  SampleTime=-1
  Unit Delay1 : UnitDelay  SampleTime=-1
  u(k) : Outport
  wires:
  Gain10/1 -> Product2/1
  r(k)/1 -> Sum3/1  "r(k)"
  y(k)/1 -> Sum3/2  "y(k)"
  Sum3/1 -> Compare To Zero2/1, Gain4/1, Gain10/1
  Saturation/1 -> u(k)/1, Sum7/2  "u(k)"
  Sum/1 -> Sum7/1, Saturation/1
  Product2/1 -> Sum2/1
  Unit Delay1/1 -> Product2/2
  Gain4/1 -> Sum/1
  Data Type Conversion/1 -> Unit Delay1/1
  Unit Delay/1 -> Sum2/2
  Compare To Zero4/1 -> Logical Operator3/1
  Compare To Zero2/1 -> Logical Operator/1
  Logical Operator1/1 -> Data Type Conversion/1
  Sum2/1 -> Sum/2, Compare To Zero1/1, Subtract1/1, Subtract/1, Unit Delay/1
  Logical Operator3/1 -> Logical Operator2/1
  Logical Operator/1 -> Logical Operator2/2
  Constant/1 -> Subtract/2
  Subtract/1 -> Compare To Zero4/1
  Constant1/1 -> Subtract1/2
  Subtract1/1 -> Compare To Zero5/1
  Compare To Zero5/1 -> Logical Operator3/2
  Compare To Zero1/1 -> Logical Operator/2
  Logical Operator2/1 -> Logical Operator1/2
  Sum7/1 -> Compare To Zero/1
  Compare To Zero/1 -> Logical Operator1/1

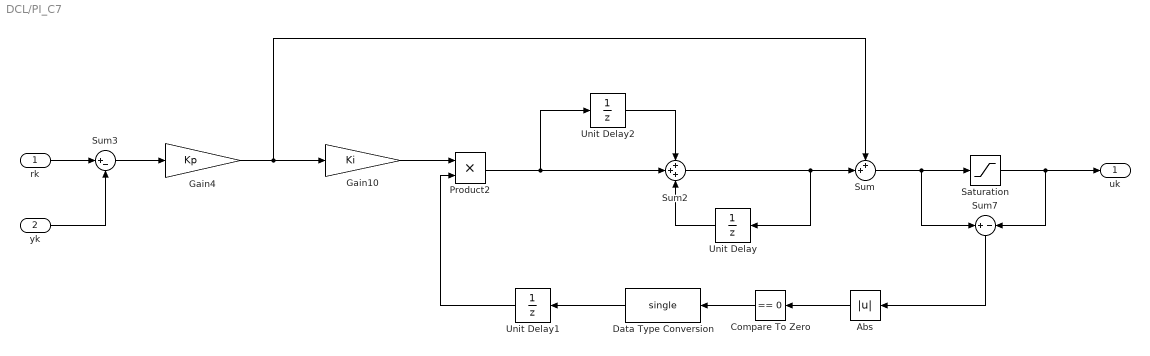
== system DCL/PI_C7 ==
  rk : Inport
  yk : Inport  Port=2
  Abs : Abs
  Compare To Zero : simulink/Logic and Bit Operations/Compare To Zero  relop===  OutDataTypeStr=uint8  ZeroCross=off
  Data Type Conversion : DataTypeConversion  OutDataTypeStr=single
  Gain10 : Gain  Gain=Ki
  Gain4 : Gain  Gain=Kp
  Product2 : Product  RndMeth=Zero
  Saturation : Saturate  UpperLimit=Uc_max  LowerLimit=Uc_min
  Sum : Sum  Inputs=++|
  Sum2 : Sum  Inputs=+++
  Sum3 : Sum  Inputs=|+-
  Sum7 : Sum  Inputs=+|-
  Unit Delay : UnitDelay  SampleTime=-1
  Unit Delay1 : UnitDelay  SampleTime=-1
  Unit Delay2 : UnitDelay  SampleTime=-1
  uk : Outport
  wires:
  Unit Delay2/1 -> Sum2/1
  Sum2/1 -> Sum/2, Unit Delay/1
  Compare To Zero/1 -> Data Type Conversion/1
  Gain10/1 -> Product2/1
  rk/1 -> Sum3/1
  Gain4/1 -> Gain10/1, Sum/1
  Unit Delay1/1 -> Product2/2
  Unit Delay/1 -> Sum2/3
  yk/1 -> Sum3/2
  Sum3/1 -> Gain4/1
  Sum/1 -> Saturation/1, Sum7/1
  Product2/1 -> Sum2/2, Unit Delay2/1
  Saturation/1 -> Sum7/2, uk/1
  Data Type Conversion/1 -> Unit Delay1/1
  Abs/1 -> Compare To Zero/1
  Sum7/1 -> Abs/1

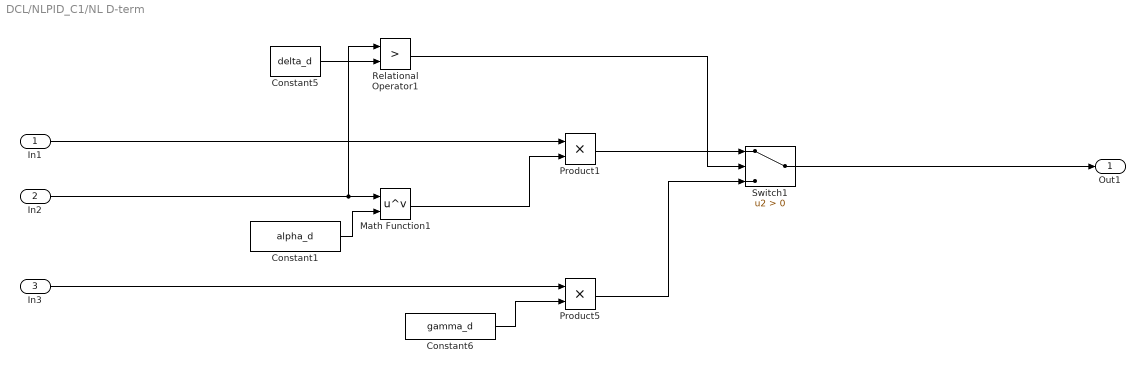
== system DCL/NLPID_C1/NL D-term ==
  In1 : Inport
  In2 : Inport  Port=2
  In3 : Inport  Port=3
  Constant1 : Constant  Value=alpha_d  OutDataTypeStr=single  SampleTime=T
  Constant5 : Constant  Value=delta_d  OutDataTypeStr=single  SampleTime=T
  Constant6 : Constant  Value=gamma_d  OutDataTypeStr=single  SampleTime=T
  Math Function1 : Math  Operator=pow  OutputSignalType=real  SaturateOnIntegerOverflow=on
  Product1 : Product  OutDataTypeStr=single  LockScale=on
  Product5 : Product  OutDataTypeStr=single  LockScale=on
  Relational Operator1 : RelationalOperator  Operator=>  OutDataTypeStr=boolean  RndMeth=Nearest  InputSameDT=on
  Switch1 : Switch  Criteria=u2 > Threshold
  Out1 : Outport
  wires:
  Constant5/1 -> Relational Operator1/2
  Switch1/1 -> Out1/1
  In1/1 -> Product1/1
  In3/1 -> Product5/1
  In2/1 -> Math Function1/1, Relational Operator1/1
  Constant1/1 -> Math Function1/2
  Product5/1 -> Switch1/3
  Product1/1 -> Switch1/1
  Relational Operator1/1 -> Switch1/2
  Math Function1/1 -> Product1/2
  Constant6/1 -> Product5/2

== system DCL/NLPID_C1/NL I-term ==
  In1 : Inport
  In2 : Inport  Port=2
  In3 : Inport  Port=3
  Constant1 : Constant  Value=alpha_i  OutDataTypeStr=single  SampleTime=T  LockScale=on
  Constant5 : Constant  Value=delta_i  OutDataTypeStr=single  SampleTime=T  LockScale=on
  Constant6 : Constant  Value=gamma_i  OutDataTypeStr=single  SampleTime=T  LockScale=on
  Math Function1 : Math  Operator=pow  OutputSignalType=real  SaturateOnIntegerOverflow=on
  Product1 : Product  OutDataTypeStr=single  InputSameDT=on  LockScale=on
  Product5 : Product  OutDataTypeStr=single  InputSameDT=on  LockScale=on
  Relational Operator1 : RelationalOperator  Operator=>  OutDataTypeStr=boolean  RndMeth=Nearest  InputSameDT=on
  Switch1 : Switch  Criteria=u2 > Threshold
  Out1 : Outport
  wires:
  Constant5/1 -> Relational Operator1/2
  Switch1/1 -> Out1/1
  Constant6/1 -> Product5/2
  Math Function1/1 -> Product1/2
  Relational Operator1/1 -> Switch1/2
  Product1/1 -> Switch1/1
  Product5/1 -> Switch1/3
  Constant1/1 -> Math Function1/2
  In2/1 -> Math Function1/1, Relational Operator1/1
  In3/1 -> Product5/1
  In1/1 -> Product1/1

== system DCL/NLPID_C1/NL P-term ==
  In1 : Inport
  In2 : Inport  Port=2
  In3 : Inport  Port=3
  Constant1 : Constant  Value=alpha_p  OutDataTypeStr=single  SampleTime=T  LockScale=on
  Constant5 : Constant  Value=delta_p  OutDataTypeStr=single  SampleTime=T  LockScale=on
  Constant6 : Constant  Value=gamma_p  OutDataTypeStr=single  SampleTime=T  LockScale=on
  Math Function1 : Math  Operator=pow  OutputSignalType=real  SaturateOnIntegerOverflow=on
  Product1 : Product  OutDataTypeStr=single  InputSameDT=on  LockScale=on
  Product5 : Product  OutDataTypeStr=single  InputSameDT=on  LockScale=on
  Relational Operator1 : RelationalOperator  Operator=>  OutDataTypeStr=boolean  RndMeth=Nearest  InputSameDT=on
  Switch1 : Switch  Criteria=u2 > Threshold  OutDataTypeStr=single  InputSameDT=on
      settings: LockScale=on
  Out1 : Outport  LockScale=on
  wires:
  Constant5/1 -> Relational Operator1/2
  Switch1/1 -> Out1/1
  Constant6/1 -> Product5/2
  Math Function1/1 -> Product1/2
  Relational Operator1/1 -> Switch1/2
  Product1/1 -> Switch1/1
  Product5/1 -> Switch1/3
  Constant1/1 -> Math Function1/2
  In2/1 -> Math Function1/1, Relational Operator1/1
  In3/1 -> Product5/1
  In1/1 -> Product1/1

== system DCL/NLPID_C1/Pre-conditioning ==
  error : Inport
  Abs1 : Abs  OutDataTypeStr=single
  Data Type Conversion2 : DataTypeConversion  OutDataTypeStr=single
  Sign1 : Signum
  sign(e) : Outport
  mod(e) : Outport  Port=2
  e : Outport  Port=3
  wires:
  Data Type Conversion2/1 -> sign(e)/1
  error/1 -> Sign1/1, Abs1/1, e/1
  Abs1/1 -> mod(e)/1
  Sign1/1 -> Data Type Conversion2/1
